simulink model "Esm"  (R2025b)
settings: Solver=FixedStepDiscrete  StartTime=0.0  StopTime=0.01  FixedStep=0.001  RelTol=1e-3
settings Model: Creator=leeyj  LastModifiedBy=leeyj

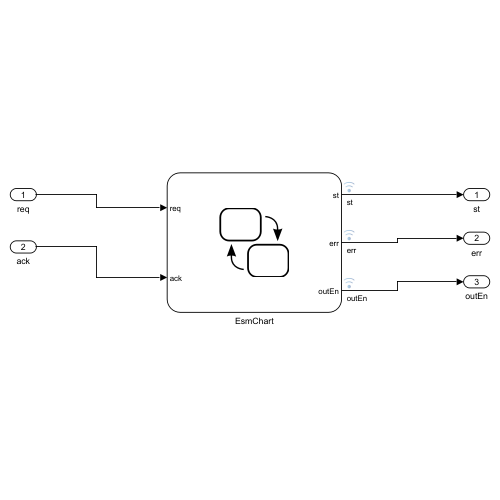
[thumbnail: Simulink's stored preview of the top-level diagram]
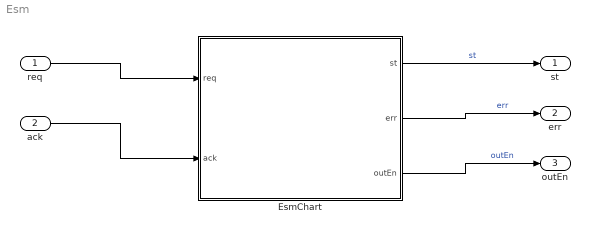
== system Esm ==
  req : Inport  OutDataTypeStr=uint8  Interpolate=off
  ack : Inport  Port=2  OutDataTypeStr=boolean  Interpolate=off
  EsmChart : Stateflow chart  TreatAsAtomicUnit=on
  st : Outport
  err : Outport  Port=2
  outEn : Outport  Port=3
  wires:
  req/1 -> EsmChart/1(req)
  ack/1 -> EsmChart/2(ack)
  EsmChart/1(st) -> st/1  "st"
  EsmChart/2(err) -> err/1  "err"
  EsmChart/3(outEn) -> outEn/1  "outEn"

== stateflow chart Esm/EsmChart ==
  settings: updateMethod=DISCRETE  sampleTime=0.001
  state Al
    during:
    err = err && !ack;
    state Init
      entry: st = 1; outEn = 0;
      during:
      err = err || (req != 0 && req != st);
    state PreOp
      entry: st = 2; outEn = 0;
      during:
      err = err || (req != 0 && req != st);
    state SafeOp
      entry: st = 4; outEn = 0;
      during:
      err = err || (req != 0 && req != st);
    state Op
      entry: st = 8; outEn = 1;
      during:
      err = err || (req != 0 && req != st);
    (default) -> Init
    Init -> PreOp : [req == 2 && !err]
    PreOp -> SafeOp [order 2] : [req == 4 && !err]
    SafeOp -> Op [order 3] : [req == 8 && !err]
    PreOp -> Init [order 1] : [req == 1]
    SafeOp -> PreOp [order 2] : [req == 2 && !err]
    Op -> SafeOp [order 3] : [req == 4 && !err]
    SafeOp -> Init [order 1] : [req == 1]
    Op -> Init [order 1] : [req == 1]
    Op -> PreOp [order 2] : [req == 2 && !err]
  (default) -> Al
  data: req input uint8; ack input boolean; st output uint8 =1; err output boolean; outEn output boolean
  data req settings: description=요청 상태 코드. 0 = 요청 없음, 1/2/4/8 = Init/PreOp/SafeOp/Op
  data ack settings: description=오류 해제
  data st settings: description=현재 상태 코드 1/2/4/8
  data err settings: description=오류 표시
  data outEn settings: description=출력 활성 = (st == 8)
